simulink model "eight"  (R2020b)
settings: Solver=VariableStepAuto  StartTime=0.0  StopTime=10.0  RelTol=1e-3
settings Model: Creator=USER  LastModifiedBy=USER

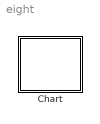
== system eight ==
  Chart : Stateflow chart  TreatAsAtomicUnit=on

== stateflow chart eight/Chart ==
  state GroundFloor
    entry:
    status=1;
    during:
    CurrentFloor=0;
    FloorCheck(CurrentFloor);
    exit:
    status=0;
  state FirstFloor
    entry:
    status=1;
    during:
    CurrentFloor=1;
    FloorCheck(CurrentFloor);
    exit:
    status=0;
  state Alarm
    (default) -> (junction 11) : % Alarm Loop
        | {alarmStatus=fire;}
    (junction 11) -> (junction 13)
    (junction 12) -> (junction 7) [order 2] : [alarmStatus==1]{send(off);}
    (junction 13) -> (junction 12) [order 1] : [1]
    (junction 12) -> (junction 3) [order 1] : [alarmStatus==0]{send(on);}
    (junction 7) -> (junction 2)
    (junction 13) -> (junction 8) [order 2]
    (junction 2) -> (junction 3)
  state SecondFloor
    entry:
    status=1;
    during:
    CurrentFloor=2;
    FloorCheck(CurrentFloor);
    exit:
    status=0;
    after(1,sec);
  state ThirdFloor
    entry:
    status=1;
    during:
    CurrentFloor=3;
    FloorCheck(CurrentFloor);
    exit:
    status=0;
    after(1,sec);
  state FourthFloor
    entry:
    status=1
    during:
    CurrentFloor=4;
    FloorCheck(CurrentFloor);
    exit:
    status=0;
  state FifthFloor
    entry:
    status=1;
    during:
    CurrentFloor=5;
    FloorCheck(CurrentFloor);
    exit:
    status=0;
  (default) -> GroundFloor
  GroundFloor -> FirstFloor : up
  FirstFloor -> GroundFloor [order 2] : down
  FirstFloor -> SecondFloor [order 1] : up
  SecondFloor -> FirstFloor [order 2] : down
  SecondFloor -> ThirdFloor [order 1] : up
  ThirdFloor -> SecondFloor [order 2] : down
  ThirdFloor -> FourthFloor [order 1] : up
  FourthFloor -> ThirdFloor [order 1] : down
  FourthFloor -> FifthFloor [order 2] : up
  FifthFloor -> FourthFloor : down
